simulink model "actionExecHier"  (Simulink 7.2)
settings: Solver=ode45  StartTime=0.0  StopTime=10  RelTol=1e-3
libraries: simulink x4
settings Model: Creator=jrivitus  LastModifiedBy=jrivitus
settings OptimizationCC: EfficientMapNaN2IntZero=off

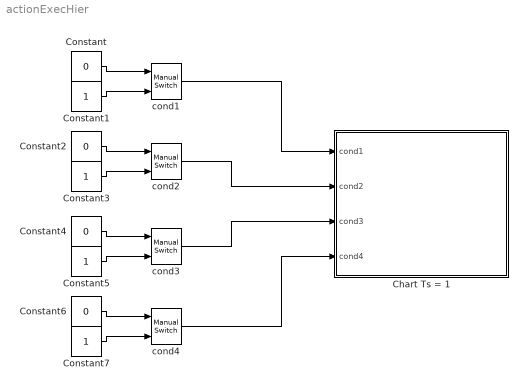
== system actionExecHier ==
  Chart Ts = 1 : Stateflow chart
  Constant{,2,4,6} (4 alike) : Constant  Value=0  OutDataType=sfix(16)  OutScaling=2^0
  Constant{1,3,5,7} (4 alike) : Constant  OutDataType=sfix(16)  OutScaling=2^0
  cond1 : simulink/Signal Routing/Manual Switch  SystemSampleTime=-1  sw=0  action=0  varsize=off
  cond2 : simulink/Signal Routing/Manual Switch  SystemSampleTime=-1  sw=1  action=0  varsize=off
  cond3 : simulink/Signal Routing/Manual Switch  SystemSampleTime=-1  sw=1  action=0  varsize=off
  cond4 : simulink/Signal Routing/Manual Switch  SystemSampleTime=-1  sw=1  action=0  varsize=off
  wires:
  Constant/1 -> cond1/1
  Constant1/1 -> cond1/2
  Constant2/1 -> cond2/1
  Constant3/1 -> cond2/2
  Constant4/1 -> cond3/1
  Constant5/1 -> cond3/2
  Constant6/1 -> cond4/1
  Constant7/1 -> cond4/2
  cond1/1 -> Chart Ts = 1/1(cond1)
  cond2/1 -> Chart Ts = 1/2(cond2)
  cond3/1 -> Chart Ts = 1/3(cond3)
  cond4/1 -> Chart Ts = 1/4(cond4)

== stateflow chart Chart Ts = 1 ==
  settings: updateMethod=DISCRETE  sampleTime=1
  state A
    during: printf("actA1\n");
    exit: printf("actA2\n");
    state A1
      during: printf("actA3\n");
      exit: printf("actA4\n");
    state A2
    (default) -> A1
    A1 -> A2 : [cond3]
    A2 -> A1 : [cond4]
  state C
  state B
    during: printf("actB1\n");
    state B1
      during: printf("actB3\n");
    state B2
    (default) -> B1 : {printf("actB2\n");}
    B1 -> B2 : [cond3]
    B2 -> B1 : [cond4]
  (default) -> A : {printf("\nSimulation started\n\n");}
  A -> (junction 10)
  (junction 10) -> C [order 2] : [cond2]
      | {printf("act2\n");}
  (junction 10) -> B [order 1] : [cond1]
      | {printf("act1\n");}
  data: cond1 input double; cond2 input double; cond3 input double; cond4 input double
